simulink model "SUPERVISOR_GLOBAL"  (R2024b)
settings: Solver=VariableStepAuto  StartTime=0.0  StopTime=10.0  RelTol=1e-3
settings Model: Creator=ribei  LastModifiedBy=ribei
settings ConfigComp: PLC_TargetIDE=codesys23  PLC_MultiTBSigbuilderTimeRange=off  PLC_FoldFBCallOutputVar=off  PLC_RemoveUnusedSSMethodCallArguments=off  PLC_UseCallOutputArgSyntax=off  PLC_EnableUnsignedAndDoubleTypes=off  PLC_EnableUDTSplitting=off  PLC_MaxFieldsInUDT=500  PLC_InlineEnumCastFunction=off

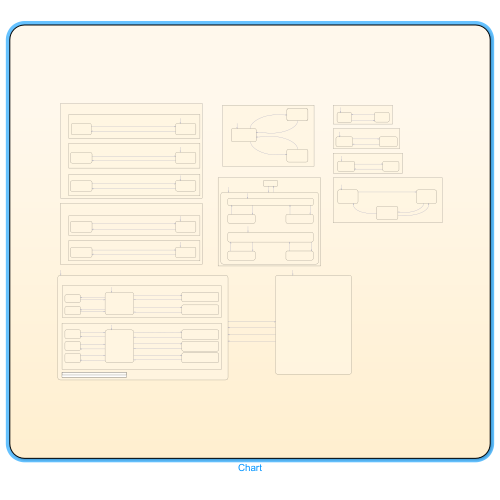
[thumbnail: Simulink's stored preview of the top-level diagram]
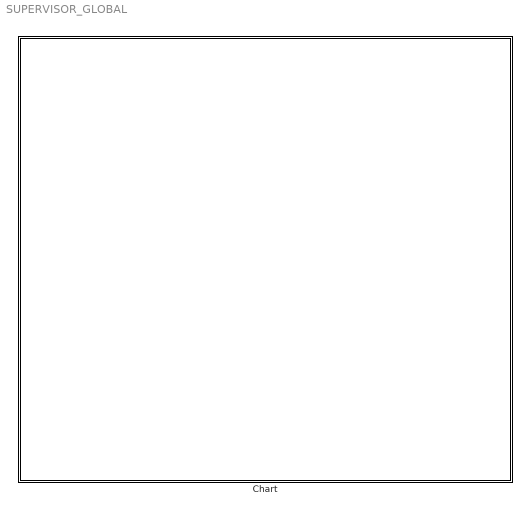
== system SUPERVISOR_GLOBAL ==
  Chart : Stateflow chart  TreatAsAtomicUnit=on

== stateflow chart SUPERVISOR_GLOBAL/Chart ==
  state FRENOS [group]
    state FRENO_IZAJE [group]
      state FRENO_IZAJE_OFF
        entry:
        BRK_h=1;
        freno_activo=0;
      state FRENO_IZAJE_ON
        entry:
        BRK_h=0;
        freno_izaje_activo=1;
      (default) -> FRENO_IZAJE_ON
      FRENO_IZAJE_OFF -> FRENO_IZAJE_ON : [(abs(whm)<=whm_min && dlh_ref_man==0 && op_mode==1) || falla_E~=0]
      FRENO_IZAJE_ON -> FRENO_IZAJE_OFF : [(Thm_disp && (dlh_ref_manual~=0 || boton_freno_izaje==1) || op_mode==0) && falla_E==0]
    state FRENO_CARRO [group]
      state FRENO_CARRO_ON
        entry:
        BRK_t=0;
        freno_carro_activo=1;
      state FRENO_CARRO_OFF
        entry:
        BRK_t=1;
        freno_carro_activo=0;
      (default) -> FRENO_CARRO_ON
      FRENO_CARRO_OFF -> FRENO_CARRO_ON : [(abs(wtm)<=wtm_min && dxt_ref_man==0 && op_mode==1) || falla_E~=0]
      FRENO_CARRO_ON -> FRENO_CARRO_OFF : [(Ttm_disp && (dxt_ref_manual~=0 || freno_manual_carro==1) || op_mode==0) && falla_E==0]
    state FRENO_EMERGENCIA [group]
      state FRENO_EM_ON
        entry:
        BRK_hE=0;
      state FRENO_EM_OFF
        entry:
        BRK_hE=1;
      (default) -> FRENO_EM_ON
      FRENO_EM_OFF -> FRENO_EM_ON : [grua_on==0 || falla_E~=0]
      FRENO_EM_ON -> FRENO_EM_OFF : [grua_on==1 && falla_E==0]
  state TWISTLOCKS [group]
    state ACT_TLK
      entry:
      TLK=1;
      c=-obst(xtd+p1)*p2/p3;
      CARGA=1;
    state VERIFICAR
      entry:
      c=0;
    state DES_TLK
      entry:
      TLK=0;
      c=obst(xtd+p1)*p2/p3;
      CARGA=0;
    VERIFICAR -> ACT_TLK [order 1] : [Sens_cont==1 && TLK_act==1 && op_mode==1 && LOAD == 0]
    ACT_TLK -> VERIFICAR
    (default) -> VERIFICAR
    DES_TLK -> VERIFICAR
    VERIFICAR -> DES_TLK [order 2] : [Sens_cont==1 && TLK_act==1 && op_mode==1 && LOAD == 0]
  state VIVO [group]
    state TALKING
      entry:
      alive==1;
    state LISTENING
      entry:
      alive=0;
    (default) -> LISTENING
    TALKING -> LISTENING : [after(500,msec)]
    LISTENING -> TALKING : [after(10,msec)]
  state CONTROL BALANCEO [group]
    state BALANCEO_ON
      entry:
      bal_control=1;
    state BALANCEO_OFF
      entry:
      bal_control=0;
    (default) -> BALANCEO_ON
    BALANCEO_ON -> BALANCEO_OFF : [~balaneceo_on || falla_E~=0]
    BALANCEO_OFF -> BALANCEO_ON : [balanceo_on]
  state TENSION CABLE IZAJE [group]
    state TENSO
      entry:
      cable_tenso=1;
    state FLOJO
      entry:
      cable_tenso=0;
    (default) -> TENSO
    TENSO -> FLOJO : [Fhw < Fhw_min]
    FLOJO -> TENSO : [Fhw >= Fhw_min]
  state SOBREVELOCIDAD [group]
    state STANDBY
    state ON
      state CARRO
        during:
        dxt_sp=dxt_ref_man;
      state SOBRE_dxt_MAX
        entry:
        dxt_sp=dxt_max;
      state SOBRE_dxt_MIN
        entry:
        dxt_sp=dxt_min;
      state IZAJE
        during:
        dhl_sp=dhl_ref_man;
      state SOBRE_dhl_MAX
        entry:
        dhl_sp=dhl_max
      state SOBRE_dhl_MIN
        entry:
        dhl_sp=dhl_min
      (default) -> SOBREVELOCIDAD.ON.CARRO [order 1]
      SOBRE_dxt_MIN -> SOBREVELOCIDAD.ON.CARRO : [dxt_sp >= dxt_min]
      SOBREVELOCIDAD.ON.CARRO -> SOBRE_dxt_MIN [order 2] : [dxt_sp < dxt_min]
      SOBRE_dxt_MAX -> SOBREVELOCIDAD.ON.CARRO : [dxt_sp <= dxt_max]
      SOBREVELOCIDAD.ON.CARRO -> SOBRE_dxt_MAX [order 1] : [dxt_sp > dxt_max]
      (default) -> SOBREVELOCIDAD.ON.IZAJE [order 2]
      SOBRE_dhl_MIN -> SOBREVELOCIDAD.ON.IZAJE : [dhl_sp >= dhl_min]
      SOBREVELOCIDAD.ON.IZAJE -> SOBRE_dhl_MIN [order 2] : [dhl_sp < dhl_min]
      SOBRE_dhl_MAX -> SOBREVELOCIDAD.ON.IZAJE : [dhl_sp <= dhl_max]
      SOBREVELOCIDAD.ON.IZAJE -> SOBRE_dhl_MAX [order 1] : [dhl_sp > dhl_max]
    STANDBY -> ON : [aceptar_carga==1]
    ON -> STANDBY : [TLK==1 && aceptar_carga==0]
    (default) -> ON
  state DETECCION SOBRECARGA [group]
    state NORMAL
      entry:
      sobrecarga=0;
      BRK_h=1;
      BRK_hE=1;
    state SOBRECARGA
      entry:
      sobrecarga=1;
      BRK_h=0;
      BRK_hE=0;
    state LIBERAR_CARGA
      entry:
      sobrecarga=0;
      BRK_h=1;
      BRK_hE=1;
    (default) -> NORMAL
    NORMAL -> DETECCION.SOBRECARGA : [cable_tenso && (Mc > Mc_max) && aceptar_carga==1]
    LIBERAR_CARGA -> DETECCION.SOBRECARGA [order 1] : [dhl_ref_man < 0]
    DETECCION.SOBRECARGA -> LIBERAR_CARGA : [dhl_ref_man > 0]
    LIBERAR_CARGA -> NORMAL [order 2] : [cable_tenso == 0]
  state FINALES DE CARRERA [group]
    state FIN_CARRERA_CARRO [group]
      state PARAR_CARRO
        entry:
        op_mode=1;
        parar_carro=1;
      state MOVER_CARRO
        entry:
        parar_carro=0;
      (default) -> MOVER_CARRO
      FINALES.FIN_CARRERA_CARRO.PARAR_CARRO -> MOVER_CARRO : [whm<=0.3]
      MOVER_CARRO -> FINALES.FIN_CARRERA_CARRO.PARAR_CARRO : [(FC_DER==1 && dx_ref<0) || (FC_IZQ==1 && dx_ref>0)]
    state FIN_CARRERA_IZAJE [group]
      state MOVER_CARGA
        entry:
        parar_carga=0;
      state PARAR_CARGA
        entry:
        op_mode=1;
        parar_carga=1;
      (default) -> MOVER_CARGA
      PARAR_CARGA -> MOVER_CARGA : [whm<=0.3]
      MOVER_CARGA -> PARAR_CARGA : [(FC_SUP==1 && dlh_ref<0) || (FC_INF && dlh_ref>0)]
  state MODO_MANUAL
    entry:
    op_mode=1;
    state CARRO [group]
      state DIST_FDC_IZQ
        during:
        dxt_ref=limitar_ac_x(dxt_sp*(30+xtd)/11);
      state CARRO_ON
        during:
        dxt_ref=limitar_vel_x(dxt_sp);
      state PARAR_CARRO
        entry:
        dxt_ref=0;
      state DIST_FDC_DER
        during:
        dxt_ref=limitar_ac_x(dxt_sp*(30-xtd)/11);
      state SOBRECARGA
        entry:
        dxt_ref=0;
      (default) -> CARRO_ON
      CARRO_ON -> DIST_FDC_IZQ [order 1] : [dxt <= -19  && dxt_ref_man < 0 && parar_carro == 0]
      CARRO_ON -> MODO_MANUAL.CARRO.PARAR_CARRO [order 3] : [parar_carro]
      DIST_FDC_IZQ -> CARRO_ON : [(dxt > -19 && dxt_ref_man > 0) || parar_carro == 1 ]
      MODO_MANUAL.CARRO.PARAR_CARRO -> CARRO_ON : [~parar_carro]
      CARRO_ON -> DIST_FDC_DER [order 2] : [dxt >= 39  && dxt_ref_man > 0 && parar_carro == 0]
      CARRO_ON -> MODO_MANUAL.CARRO.SOBRECARGA [order 4] : [sobrecarga]
      MODO_MANUAL.CARRO.SOBRECARGA -> CARRO_ON : [~sobrecarga]
      DIST_FDC_DER -> CARRO_ON : [(dxt < 39 && dxt_ref_man < 0) || parar_carro == 1 ]
    state IZAJE [group]
      state PARAR_IZAJE
        entry:
        dlh_ref=0;
      state IZAJE_ON
        during:
        dlh_ref=limitar_vel_y(dlh_sp,0);
      state DIST_FDC_SUP
        during:
        dlh_ref=limitar_vel_y(dlh_sp*(lh-5)/7,0);
      state SOBRECARGA
        entry:
        dlh_ref=0;
        limitar_vel_y(0,1);
      state DIST_FDC_INF
        during:
        dlh_ref=limitar_vel_y(dlh_sp*(65-lh)/10,0);
      state ALTURA_BAJA
        during:
        dlh_ref=limitar_vel_y(dlh_sp,0)*0.1;
        exit:
        limitar_vel_y(dlh_ref,1);
      state CABLE_TENSO
        entry:
        dlh_ref=-2;
      (default) -> IZAJE_ON
      IZAJE_ON -> DIST_FDC_SUP [order 1] : [lh <= 12 && dlh_ref_man < 0 && detener_izaje == 0]
      PARAR_IZAJE -> IZAJE_ON : [~parar_izaje]
      IZAJE_ON -> PARAR_IZAJE [order 3] : [parar_izaje]
      DIST_FDC_SUP -> IZAJE_ON : [(lh > 12 && dlh_ref_man > 0) || detener_izaje == 1 ]
      MODO_MANUAL.IZAJE.SOBRECARGA -> IZAJE_ON : [~sobrecarga]
      IZAJE_ON -> DIST_FDC_INF [order 2] : [lh >= 55 && dlh_ref_man > 0 && detener_izaje == 0]
      IZAJE_ON -> MODO_MANUAL.IZAJE.SOBRECARGA [order 4] : [sobrecarga]
      DIST_FDC_INF -> IZAJE_ON : [(lh < 55 && dlh_ref_man > 0) && detener_izaje == 1]
      IZAJE_ON -> ALTURA_BAJA [order 6] : [TLK==1 && aceptar_carga == 0]
      CABLE_TENSO -> IZAJE_ON : [cable_tenso]
      ALTURA_BAJA -> IZAJE_ON : [aceptar_carga == 1]
      IZAJE_ON -> CABLE_TENSO [order 5] : [~cable_tenso]
  state MODO_AUTOMATICO
    entry:
    op_mode = 0;
    it = 0;
    x_fin_consigna = destino;
    x_ini = x_td;
    y_ini = 45-lh;
    pos_ref = gen_coords(Y_c0_mod, dlh_max, x_ini, x_fin_consigna, y_ini, LOAD, Ts);
    parametros = size(pos_ref);
    Kp = 0.2;
    during:
    it = it+1;
    if (it > size(pos_ref) && abs(xt_ref - xtd) > 0.5 && it < it_fin)
    dxt_ref = Kp*(xt_ref - xtd)/2;
    dlh_ref = 0.8*(lh_ref - lh)/2;
    elseif (it <= parametros(2))
    xt_ref = pos_ref(1,it);
    lh_ref = pos_ref(2,it);
    dxt_ref = Kp*(xt_ref - xtd);
    dlh_ref = 0.30*(lh_ref - lh);
    else
    it_fin = it;
    dxt_ref = 0;
    dlh_ref = 0;
    end
  (default) -> MODO_MANUAL [order 13]
  (default) -> MODO_AUTOMATICO [order 4]
  MODO_MANUAL -> MODO_AUTOMATICO : [selec_mode == 0]
  MODO_AUTOMATICO -> MODO_MANUAL [order 1] : [FDC_DER || FDC_IZQ || FDC_SUP || FDC_INF]
  MODO_AUTOMATICO -> MODO_MANUAL [order 2] : [dxt_ref_man ~= 0 || dlh_ref_man ~= 0]
  MODO_AUTOMATICO -> MODO_MANUAL [order 3] : [selec_mode == 1]
  data: set_point function_input; vel_x function_output; set_point function_input; vel_y function_output; cargado function_input
  function vel_x = limitar_vel_x(set_point):
    | function vel_x = limitar_vel_x(set_point)
    | 
    | persistent vt_actual
    | 
    | if isempty(vt_actual)
    |     vt_actual = 0;
    | end
    | 
    |     if abs(set_point) >= vt_actual
    |         if set_point > 0
    |             vel_x = at_max * dt + vt_actual;
    |         elseif set_point < 0
    |             vel_x = -at_max * dt + vt_actual;
    |         else
    |             vel_x = vt_actual;
    |         end
    |     end
    | 
    |     if vel_x >= vt_max
    |         vel_x = vt_max;
    |     elseif vel_x <= -vt_max
    |         vel_x = -vt_max;
    |     end
    | 
    |     vt_actual = vel_x;
    | 
    | end
  function vel_y = limitar_vel_y(set_point, cargado):
    | function vel_y = limitar_vel_y(set_point, cargado)
    | 
    | persistent vt_actual
    | 
    | if isempty(vt_actual)
    |     vt_actual = 0;
    | end
    | 
    |     if abs(set_point) >= vt_actual
    |         if set_point > 0
    |             vel_x = at_max * dt + vt_actual;
    |         elseif set_point < 0
    |             vel_x = -at_max * dt + vt_actual;
    |         end
    |     end
    | 
    |     if vel_x >= vt_max
    |         vel_x = vt_max;
    |     elseif vel_x <= -vt_max
    |         vel_x = -vt_max;
    |     end
    | 
    |     vt_actual = vel_x;
    | 
    | end
